simulink model "II"  (R2018a)
settings: Solver=VariableStepAuto  StartTime=0.0  StopTime=10  RelTol=1e-3
libraries: dsparch4 x1
settings Model: Creator=User  LastModifiedBy=User

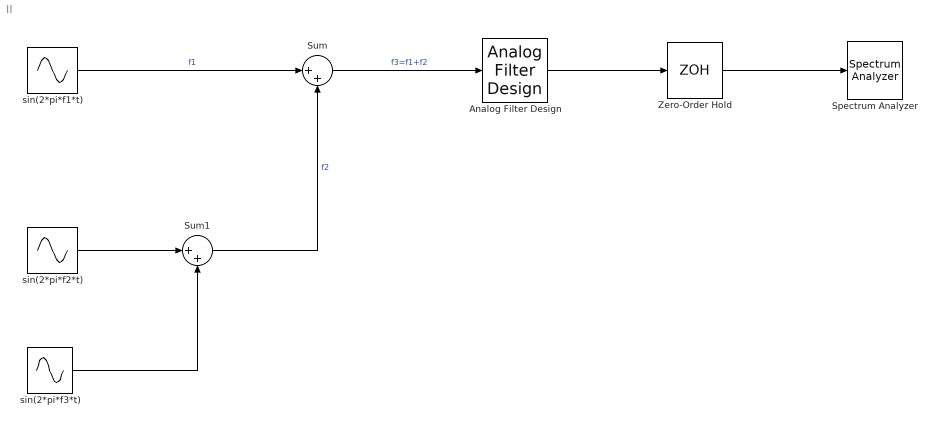
== system II ==
  Analog Filter Design : dsparch4/Analog Filter Design  method=Butterworth  filttype=Lowpass  N=8  Wlo=2*pi*200  Whi=2*pi*180  Rp=2  Rs=40
  Spectrum Analyzer : SpectrumAnalyzer
  Sum : Sum  Inputs=|++
  Sum1 : Sum  Inputs=|++
  Zero-Order Hold : ZeroOrderHold  SampleTime=0.0025
  sin(2*pi*f1*t) : Sin  Frequency=2*pi*100  SampleTime=0
  sin(2*pi*f2*t) : Sin  Frequency=2*pi*160  SampleTime=0
  sin(2*pi*f3*t) : Sin  Frequency=2*pi*1000  SampleTime=0
  wires:
  sin(2*pi*f1*t)/1 -> Sum/1  "f1"
  Sum/1 -> Analog Filter Design/1  "f3=f1+f2"
  Analog Filter Design/1 -> Zero-Order Hold/1
  Zero-Order Hold/1 -> Spectrum Analyzer/1
  sin(2*pi*f2*t)/1 -> Sum1/1
  sin(2*pi*f3*t)/1 -> Sum1/2
  Sum1/1 -> Sum/2  "f2"
